simulink model "SimHinfLin"  (R2021b)
settings: Solver=VariableStepAuto  StartTime=0.0  StopTime=9  RelTol=1e-3
undefined symbols (not defined in the file): Alatdir, Along, Blatdir, Blong, Clatdir, Clong, Dlatdir, Dlong, K, K1
libraries: simulink x1
settings Model: Creator=Daniel  LastModifiedBy=Daniel

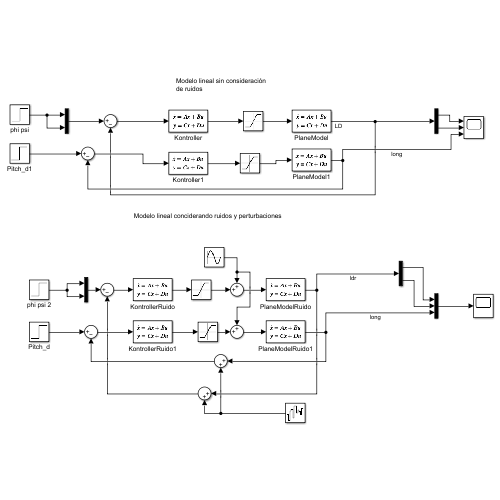
[thumbnail: Simulink's stored preview of the top-level diagram]
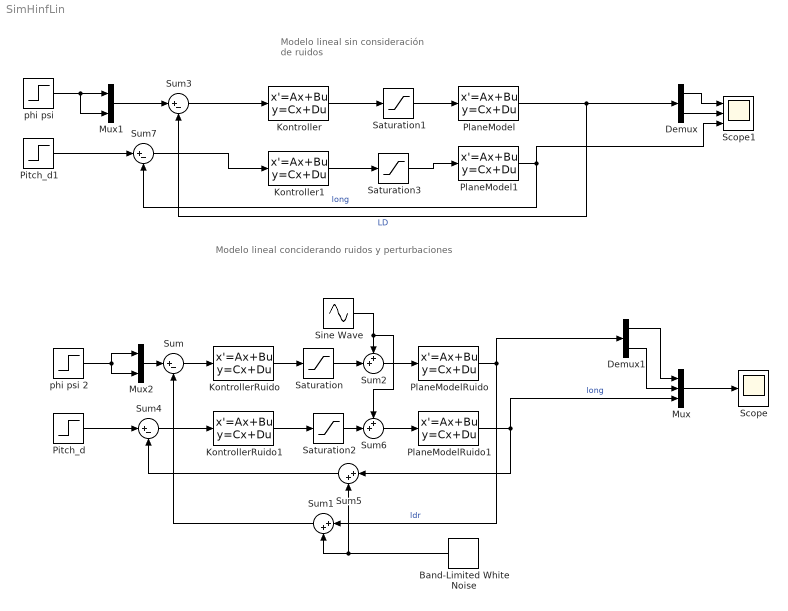
== system SimHinfLin ==
  note: Modelo lineal conciderando ruidos y perturbaciones
  note: Modelo lineal sin consideración
      | de ruidos
  Band-Limited White Noise : simulink/Sources/Band-Limited White Noise  Cov=[0.0001]  Ts=0.1  seed=[23341]
  Demux : Demux  Outputs=2
  Demux1 : Demux  Outputs=2
  Kontroller : StateSpace  A=K1.A  B=K1.B  C=K1.C  D=K1.D  InitialCondition=0
  Kontroller1 : StateSpace  A=K.A  B=K.B  C=K.C  D=K.D  InitialCondition=0
  KontrollerRuido : StateSpace  A=K1.A  B=K1.B  C=K1.C  D=K1.D  InitialCondition=0
  KontrollerRuido1 : StateSpace  A=K.A  B=K.B  C=K.C  D=K.D  InitialCondition=0
  Mux : Mux  Inputs=3
  Mux1 : Mux  Inputs=2
  Mux2 : Mux  Inputs=2
  Pitch_d : Step  After=40  SampleTime=0
  Pitch_d1 : Step  After=40  SampleTime=0
  PlaneModel : StateSpace  A=Alatdir  B=Blatdir  C=Clatdir  D=Dlatdir  InitialCondition=0
  PlaneModel1 : StateSpace  A=Along  B=Blong  C=Clong  D=Dlong  InitialCondition=0
  PlaneModelRuido : StateSpace  A=Alatdir  B=Blatdir  C=Clatdir  D=Dlatdir  InitialCondition=0
  PlaneModelRuido1 : StateSpace  A=Along  B=Blong  C=Clong  D=Dlong  InitialCondition=0
  Saturation{,1..3} (4 alike) : Saturate  UpperLimit=30  LowerLimit=-30
  Scope : Scope
  Scope1 : Scope  NumInputPorts=3
  Sine Wave : Sin  Frequency=12*pi  SampleTime=0
  Sum{,3..4,7} (4 alike) : Sum  Inputs=|+-
  Sum1 : Sum  Inputs=|++
  Sum2 : Sum  Inputs=++|
  Sum5 : Sum  Inputs=|++
  Sum6 : Sum  Inputs=++|
  phi psi : Step  Time=0  After=40  SampleTime=0
  phi psi 2 : Step  After=40  SampleTime=0
  wires:
  Mux1/1 -> Sum3/1
  PlaneModel/1 -> Sum3/2, Demux/1  "LD"
  KontrollerRuido/1 -> Saturation/1
  Saturation/1 -> Sum2/2
  Band-Limited White Noise/1 -> Sum5/2, Sum1/2
  Sum2/1 -> PlaneModelRuido/1
  Saturation1/1 -> PlaneModel/1
  PlaneModelRuido/1 -> Demux1/1, Sum1/1  "ldr"
  Kontroller/1 -> Saturation1/1
  Sum1/1 -> Sum/2
  phi psi 2/1 -> Mux2/2, Mux2/1
  Sine Wave/1 -> Sum6/1, Sum2/1
  Sum3/1 -> Kontroller/1
  Mux2/1 -> Sum/1
  phi psi/1 -> Mux1/2, Mux1/1
  Kontroller1/1 -> Saturation3/1
  Pitch_d1/1 -> Sum7/1
  Saturation2/1 -> Sum6/2
  PlaneModel1/1 -> Sum7/2, Scope1/3  "long"
  Sum7/1 -> Kontroller1/1
  Saturation3/1 -> PlaneModel1/1
  Sum6/1 -> PlaneModelRuido1/1
  Sum5/1 -> Sum4/2
  Pitch_d/1 -> Sum4/1
  Sum4/1 -> KontrollerRuido1/1
  KontrollerRuido1/1 -> Saturation2/1
  PlaneModelRuido1/1 -> Mux/3, Sum5/1  "long"
  Demux/1 -> Scope1/1
  Demux/2 -> Scope1/2
  Demux1/1 -> Mux/1
  Demux1/2 -> Mux/2
  Sum/1 -> KontrollerRuido/1
  Mux/1 -> Scope/1
